simulink model "fin_long_curs2"  (R2019a)
settings: Solver=VariableStepAuto  StartTime=0.0  StopTime=100  RelTol=1e-3
values from neighbouring files (symbols this model uses):
  c1 = 743    [scr1.m]
  C_d1 = c_dl1    [scr1.m]
  C_d3 = c_dl_3    [scr1.m]
  C_n1 = c_np1    [scr1.m]
  C_n3 = c_np_3    [scr1.m]
  Ca = 1.19    [scr1.m]
  d12 = conv(d1,d2)    [scr1.m]
  g = 9.8    [scr1.m]
  kr = 0.00026918    [scr1.m]
  M = 1500    [scr1.m]
  n4 = c1/(T*tau1)    (= 3715)    [scr1.m]
  T = 1    [scr1.m]
  tau1 = 0.2    [scr1.m]
  v = 25    [scr1.m]
undefined symbols (not defined in the file or in its folder): c7_dem, c7_num, ci6
settings Model: Creator=hvarol1  LastModifiedBy=Ya
settings DataIOCC: ReturnWorkspaceOutputs=off
settings DebuggingCC: ArithmeticOperatorsInVariantConditions=warning

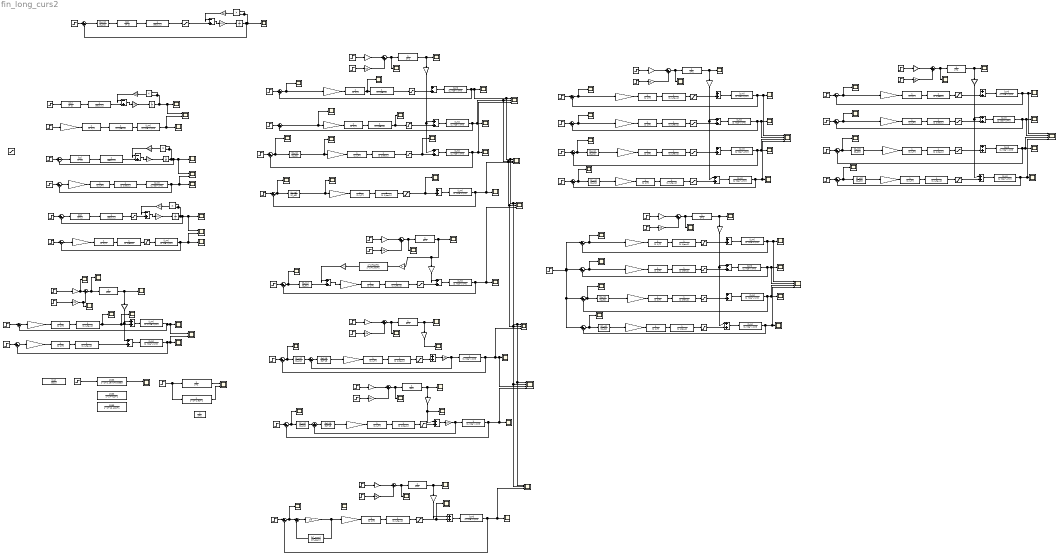
== system fin_long_curs2 ==
  Gain{,1..2,6,30,52} (6 alike) : Gain  Gain=1/M
  Gain{10,16,20,29,32,36,45,55,58} (9 alike) : Gain  Gain=M*g
  Gain{11,17,21,27,33,37,46,56,59} (9 alike) : Gain  Gain=-1
  Gain{3..4,7,12,18,22,28,31,34,38,47,57,60} (13 alike) : Gain  Gain=Ca
  Gain13 : Gain
  Gain14 : Gain  Gain=kr
  Gain{5,8..9,15,19,24..26,35,39..44,48..51,53..54,61..64} (25 alike) : Gain  Gain=c1/(T*tau1)
  Gain23 : Gain  Gain=ci6
  Integrator{,1..3} (4 alike) : Integrator
  Product{1..4} (4 alike) : Product
  Saturation{1,16..19} (5 alike) : Saturate  UpperLimit=16000  LowerLimit=-16000
  Saturation{3..15,20..24} (18 alike) : Saturate  UpperLimit=3500  LowerLimit=-3500
  Saturation2 : Saturate  UpperLimit=10000  LowerLimit=-10000
  Scope{1..4,6..10,12..19,21..25,27,29,32..34,36..41,43..48,50..54,56..64,66..75,77..79,81..93,95..96} (81 alike) : Scope
  Scope{5,11,28,30,35,42} (6 alike) : Scope  NumInputPorts=2
  Scope{20,26,31,49,55} (5 alike) : Scope  NumInputPorts=3
  Scope{65,76,80,94} (4 alike) : Scope  NumInputPorts=4
  Step{,3,9,38} (4 alike) : Step  SampleTime=0
  Step{1..2,4..5,7,10,13,16..19,24..27,30..32,35..37,39..40} (23 alike) : Step  After=25  SampleTime=0
  Step{6,11,14,22,28,33,41,43} (8 alike) : Step  After=100  SampleTime=0
  Step{8,12,15,23,29,34,42,44} (8 alike) : Step  After=0.1  SampleTime=0
  Step20 : Step  Time=300  After=100  SampleTime=0
  Step21 : Step  Time=300  After=0.1  SampleTime=0
  Step45 : Step  Time=50  Before=25  After=35  SampleTime=0
  Sum{1..2,7,28} (4 alike) : Sum  Inputs=|-+
  Sum{8,10,12..14,16,18,20,22..23,25,29..30,32,34,36,38..39,41..42,44,46,48,50,52,54,56,58..59,61,63,65} (32 alike) : Sum  Inputs=|++
  Sum{3..6,9,11,15,17,19,21,24,26..27,31,33,35,37,40,43,45,47,49,51,53,55,57,60,62,64,66} (30 alike) : Sum  Inputs=|+-
  Transfer Fcn{1,7,20,33,60,67,98,108,112} (9 alike) : TransferFcn  Numerator=[C_n1]  Denominator=[C_d1]
  Transfer Fcn{2,4,10,52} (4 alike) : TransferFcn  Denominator=[tau1 1]
  Transfer Fcn100 : TransferFcn  Numerator=[6 18]  Denominator=[5 15]
  Transfer Fcn{6,21,28,39,46,48,53,80,99,101} (10 alike) : TransferFcn  Denominator=[1 1]
  Transfer Fcn{11,14,17,26,30,37,40,49,54,57,61,64,69,71,74,77,81,84,88,92,95,102,105,109,113} (25 alike) : TransferFcn  Denominator=[1 1/T]
  Transfer Fcn{12,15,18,31,34,38,44,50,55,58,62,65,70,72,75,78,82,85,89,93,96,103,106,110,114} (25 alike) : TransferFcn  Denominator=[1 1/tau1]
  Transfer Fcn{16,19,35,45,56,59,63,66,68,73,76,79,83,86,90,94,104,107,111,115} (20 alike) : TransferFcn  Numerator=[1/M]  Denominator=[1 ((Ca*v)/M)]
  Transfer Fcn13 : TransferFcn  Numerator=[1/M]  Denominator=[1 (Ca*v/M)]
  Transfer Fcn22 : TransferFcn  Numerator=[1 6 5]  Denominator=[1 1.8 1]
  Transfer Fcn23 : TransferFcn  Numerator=[1583]  Denominator="[1 2.167  0.8333]"
  Transfer Fcn24 : TransferFcn  Numerator=[n4]  Denominator=[d12]
  Transfer Fcn25 : TransferFcn  Numerator=[1583]  Denominator="[1 41  1]"
  Transfer Fcn27 : TransferFcn  Numerator=[1583]  Denominator="[1 12.48  1]"
  Transfer Fcn29 : TransferFcn  Denominator=[1 1.8 1]
  Transfer Fcn{3,5,9,51} (4 alike) : TransferFcn  Numerator=[c1]  Denominator=[T 1]
  Transfer Fcn32 : TransferFcn  Denominator=[1 ((Ca*v)/M)]
  Transfer Fcn36 : TransferFcn  Numerator=[1/M]  Denominator=[1 (2*Ca*v/M)]
  Transfer Fcn41 : TransferFcn  Numerator=[1/M]  Denominator=[1 (Ca*v/M)]
  Transfer Fcn42 : TransferFcn  Numerator=[6 18]  Denominator=[5 15]
  Transfer Fcn43 : TransferFcn  Numerator=[1 0]  Denominator=[1 1]
  Transfer Fcn47 : TransferFcn  Numerator=[c7_num]  Denominator=[c7_dem]
  Transfer Fcn8 : TransferFcn  Numerator=[C_n3]  Denominator=[C_d3]
  Transfer Fcn87 : TransferFcn  Numerator=[C_n3]  Denominator=[C_d3]
  Transfer Fcn91 : TransferFcn  Numerator=[C_n3]  Denominator=[C_d3]
  Transfer Fcn97 : TransferFcn  Denominator=[1 ((Ca*v)/M)]
  wires:
  Transfer Fcn3/1 -> Transfer Fcn4/1
  Step7/1 -> Sum5/1
  Gain6/1 -> Integrator/1
  Sum7/1 -> Gain6/1
  Product1/1 -> Gain7/1
  Integrator/1 -> Scope28/1, Scope12/1, Sum5/2, Product1/2, Product1/1
  Gain7/1 -> Sum7/1
  Sum1/1 -> Gain2/1
  Product2/1 -> Gain4/1
  Transfer Fcn9/1 -> Transfer Fcn10/1
  Transfer Fcn10/1 -> Sum1/2
  Gain4/1 -> Sum1/1
  Gain2/1 -> Integrator1/1
  Integrator1/1 -> Product2/1, Product2/2, Scope11/1, Scope2/1
  Step3/1 -> Transfer Fcn9/1
  Gain5/1 -> Transfer Fcn14/1
  Transfer Fcn14/1 -> Transfer Fcn15/1
  Sum6/1 -> Gain5/1
  Step4/1 -> Sum6/1
  Sum5/1 -> Transfer Fcn3/1
  Transfer Fcn34/1 -> Sum18/2
  Transfer Fcn38/1 -> Scope38/1, Sum20/2, Scope37/1
  Sum20/1 -> Transfer Fcn36/1
  Sum19/1 -> Gain25/1
  Transfer Fcn36/1 -> Scope35/1, Scope34/1, Sum21/2
  Step18/1 -> Sum19/1
  Gain26/1 -> Transfer Fcn37/1
  Sum18/1 -> Transfer Fcn35/1
  Step19/1 -> Sum21/1
  Transfer Fcn35/1 -> Sum19/2, Scope35/2, Scope33/1
  Step20/1 -> Gain28/1
  Gain28/1 -> Scope40/1, Sum22/2
  Gain29/1 -> Scope41/1, Sum22/1
  Sum21/1 -> Gain26/1
  Gain25/1 -> Transfer Fcn26/1
  Transfer Fcn26/1 -> Transfer Fcn34/1
  Gain27/1 -> Sum18/1, Sum20/1
  Step21/1 -> Gain29/1
  Transfer Fcn37/1 -> Transfer Fcn38/1
  Sum22/1 -> Transfer Fcn46/1, Scope39/1
  Transfer Fcn46/1 -> Gain27/1, Scope36/1
  Transfer Fcn68/1 -> Scope11/2, Scope77/1
  Gain53/1 -> Transfer Fcn71/1
  Transfer Fcn71/1 -> Transfer Fcn72/1
  Step38/1 -> Gain53/1
  Gain35/1 -> Transfer Fcn64/1
  Step27/1 -> Sum40/1
  Transfer Fcn65/1 -> Saturation6/1
  Transfer Fcn64/1 -> Scope14/1, Transfer Fcn65/1
  Transfer Fcn66/1 -> Scope80/1, Scope55/1, Scope49/1, Scope31/1, Scope20/1, Scope26/1, Scope15/1, Sum40/2
  Sum39/1 -> Transfer Fcn66/1
  Gain36/1 -> Sum41/1
  Step28/1 -> Gain38/1
  Sum42/1 -> Transfer Fcn73/1
  Transfer Fcn73/1 -> Scope80/2, Scope55/2, Scope49/2, Scope31/2, Scope20/2, Scope26/2, Scope25/1, Sum43/2
  Step30/1 -> Sum43/1
  Transfer Fcn69/1 -> Transfer Fcn70/1
  Gain39/1 -> Transfer Fcn69/1
  Transfer Fcn74/1 -> Transfer Fcn75/1
  Transfer Fcn76/1 -> Scope26/3, Scope27/1, Sum45/2
  Sum44/1 -> Transfer Fcn76/1
  Step31/1 -> Sum45/1
  Gain40/1 -> Transfer Fcn74/1
  Gain37/1 -> Sum44/1, Sum42/1
  Product3/1 -> Gain3/1
  Gain1/1 -> Integrator2/1
  Integrator2/1 -> Scope1/1, Product3/1, Product3/2, Sum4/2
  Sum2/1 -> Gain1/1
  Gain3/1 -> Sum2/1
  Transfer Fcn2/1 -> Saturation1/1
  Transfer Fcn5/1 -> Transfer Fcn2/1
  Step1/1 -> Sum4/1
  Sum4/1 -> Transfer Fcn1/1
  Transfer Fcn1/1 -> Transfer Fcn5/1
  Transfer Fcn72/1 -> Transfer Fcn68/1
  Transfer Fcn13/1 -> Sum6/2, Scope4/1, Scope28/2
  Transfer Fcn70/1 -> Saturation8/1, Scope7/1
  Gain38/1 -> Sum41/2
  Step29/1 -> Gain36/1
  Transfer Fcn7/1 -> Scope9/1, Gain40/1
  Sum45/1 -> Transfer Fcn7/1, Scope8/1
  Sum40/1 -> Gain35/1, Scope13/1
  Saturation8/1 -> Sum42/2
  Sum43/1 -> Scope6/1, Gain39/1
  Saturation6/1 -> Sum39/2
  Transfer Fcn75/1 -> Saturation3/1
  Sum41/1 -> Transfer Fcn6/1, Scope24/1
  Transfer Fcn6/1 -> Gain37/1, Scope23/1
  Saturation3/1 -> Scope10/1, Sum44/2
  Saturation1/1 -> Sum2/2
  Transfer Fcn8/1 -> Scope19/1, Gain8/1
  Saturation4/1 -> Scope16/1, Sum8/2
  Transfer Fcn11/1 -> Transfer Fcn12/1
  Step2/1 -> Sum9/1
  Gain8/1 -> Transfer Fcn11/1
  Transfer Fcn12/1 -> Saturation4/1
  Transfer Fcn16/1 -> Scope20/3, Scope17/1, Sum9/2
  Sum9/1 -> Transfer Fcn8/1, Scope18/1
  Sum8/1 -> Transfer Fcn16/1
  Sum11/1 -> Transfer Fcn20/1, Scope29/1
  Transfer Fcn19/1 -> Scope31/3, Scope22/1, Sum11/2
  Gain9/1 -> Transfer Fcn17/1
  Transfer Fcn18/1 -> Saturation5/1
  Transfer Fcn17/1 -> Transfer Fcn18/1
  Step5/1 -> Sum11/1
  Sum12/1 -> Transfer Fcn21/1, Scope32/1
  Gain12/1 -> Sum12/2
  Step6/1 -> Gain12/1
  Gain10/1 -> Sum12/1
  Step8/1 -> Gain10/1
  Sum13/1 -> Gain9/1
  Transfer Fcn20/1 -> Sum13/2
  Transfer Fcn22/1 -> Gain13/1
  Step/1 -> Transfer Fcn23/1
  Transfer Fcn23/1 -> Scope30/1
  Step9/1 -> Transfer Fcn28/1, Transfer Fcn29/1
  Transfer Fcn28/1 -> Scope42/1
  Transfer Fcn29/1 -> Scope42/2
  Sum10/1 -> Transfer Fcn19/1
  Saturation5/1 -> Sum10/2
  Gain13/1 -> Sum13/1
  Gain14/1 -> Transfer Fcn22/1
  Transfer Fcn21/1 -> Gain11/1, Gain14/1, Scope21/1
  Sum15/1 -> Scope45/1, Transfer Fcn33/1
  Transfer Fcn32/1 -> Scope49/3, Scope80/3, Scope44/1, Sum15/2
  Gain15/1 -> Transfer Fcn30/1
  Sum14/1 -> Gain/1
  Transfer Fcn30/1 -> Transfer Fcn31/1
  Step10/1 -> Sum15/1
  Sum16/1 -> Transfer Fcn39/1, Scope48/1
  Gain18/1 -> Sum16/2
  Step11/1 -> Gain18/1
  Transfer Fcn39/1 -> Scope47/1, Gain17/1
  Gain16/1 -> Sum16/1
  Step12/1 -> Gain16/1
  Gain17/1 -> Scope43/1
  Transfer Fcn33/1 -> Sum17/1
  Transfer Fcn31/1 -> Saturation9/1
  Gain/1 -> Sum17/2, Transfer Fcn32/1
  Sum17/1 -> Transfer Fcn42/1
  Saturation9/1 -> Sum14/2
  Transfer Fcn42/1 -> Gain15/1
  Transfer Fcn45/1 -> Scope55/3, Scope50/1, Sum24/2
  Gain19/1 -> Transfer Fcn40/1
  Transfer Fcn44/1 -> Saturation7/1
  Saturation7/1 -> Scope46/1, Sum23/2
  Sum23/1 -> Transfer Fcn45/1
  Transfer Fcn40/1 -> Transfer Fcn44/1
  Step13/1 -> Sum24/1
  Gain21/1 -> Sum23/1
  Sum25/1 -> Transfer Fcn48/1, Scope54/1
  Transfer Fcn48/1 -> Scope53/1, Gain21/1
  Gain20/1 -> Sum25/1
  Gain22/1 -> Sum25/2
  Step15/1 -> Gain20/1
  Step14/1 -> Gain22/1
  Sum26/1 -> Gain23/1
  Gain23/1 -> Transfer Fcn47/1, Gain19/1
  Transfer Fcn47/1 -> Sum26/2
  Sum24/1 -> Scope51/1, Sum26/1
  Transfer Fcn15/1 -> Transfer Fcn13/1
  Transfer Fcn4/1 -> Sum7/2
  Saturation13/1 -> Sum28/2
  Step16/1 -> Sum27/1
  Sum3/1 -> Transfer Fcn51/1
  Sum27/1 -> Gain24/1
  Integrator3/1 -> Scope5/1, Scope3/1, Sum3/2, Product4/2, Product4/1
  Step17/1 -> Sum3/1
  Transfer Fcn52/1 -> Saturation13/1
  Gain31/1 -> Sum28/1
  Product4/1 -> Gain31/1
  Transfer Fcn49/1 -> Transfer Fcn50/1
  Transfer Fcn51/1 -> Transfer Fcn52/1
  Gain24/1 -> Transfer Fcn49/1
  Gain30/1 -> Integrator3/1
  Saturation12/1 -> Transfer Fcn41/1
  Sum28/1 -> Gain30/1
  Transfer Fcn41/1 -> Sum27/2, Scope56/1, Scope5/2
  Transfer Fcn50/1 -> Saturation12/1
  Sum29/1 -> Transfer Fcn53/1, Scope58/1
  Gain34/1 -> Sum29/2
  Step22/1 -> Gain34/1
  Transfer Fcn53/1 -> Gain33/1, Scope57/1
  Gain32/1 -> Sum29/1
  Step23/1 -> Gain32/1
  Transfer Fcn56/1 -> Sum31/2, Scope61/1, Scope65/1
  Sum30/1 -> Transfer Fcn56/1
  Step24/1 -> Sum31/1
  Gain41/1 -> Transfer Fcn54/1
  Sum31/1 -> Gain41/1, Scope59/1
  Transfer Fcn54/1 -> Transfer Fcn55/1
  Transfer Fcn55/1 -> Saturation10/1
  Saturation10/1 -> Sum30/2
  Transfer Fcn58/1 -> Saturation11/1
  Transfer Fcn57/1 -> Transfer Fcn58/1
  Saturation11/1 -> Sum32/2
  Sum33/1 -> Gain42/1, Scope62/1
  Step25/1 -> Sum33/1
  Gain42/1 -> Transfer Fcn57/1
  Transfer Fcn59/1 -> Sum33/2, Scope64/1, Scope65/2
  Sum32/1 -> Transfer Fcn59/1
  Transfer Fcn60/1 -> Gain43/1
  Saturation14/1 -> Sum34/2
  Transfer Fcn61/1 -> Transfer Fcn62/1
  Step26/1 -> Sum35/1
  Gain43/1 -> Transfer Fcn61/1
  Transfer Fcn62/1 -> Saturation14/1
  Transfer Fcn63/1 -> Sum35/2, Scope66/1, Scope65/3
  Sum35/1 -> Transfer Fcn60/1, Scope67/1
  Sum34/1 -> Transfer Fcn63/1
  Gain44/1 -> Transfer Fcn77/1
  Step32/1 -> Sum37/1
  Transfer Fcn78/1 -> Saturation15/1
  Sum36/1 -> Transfer Fcn79/1
  Transfer Fcn77/1 -> Transfer Fcn78/1
  Saturation15/1 -> Sum36/2
  Transfer Fcn79/1 -> Sum37/2, Scope65/4, Scope60/1
  Transfer Fcn67/1 -> Gain44/1
  Sum37/1 -> Transfer Fcn67/1, Scope63/1
  Gain33/1 -> Sum36/1, Sum32/1
  Sum53/1 -> Transfer Fcn91/1, Scope74/1
  Saturation19/1 -> Sum52/2
  Transfer Fcn92/1 -> Transfer Fcn93/1
  Transfer Fcn94/1 -> Sum53/2, Scope76/4, Scope71/1
  Sum52/1 -> Transfer Fcn94/1
  Step39/1 -> Sum53/1
  Gain50/1 -> Transfer Fcn88/1
  Transfer Fcn89/1 -> Saturation18/1
  Saturation17/1 -> Sum48/2
  Sum50/1 -> Transfer Fcn90/1
  Sum51/1 -> Transfer Fcn87/1, Scope79/1
  Transfer Fcn88/1 -> Transfer Fcn89/1
  Saturation16/1 -> Sum46/2
  Transfer Fcn82/1 -> Saturation16/1
  Transfer Fcn81/1 -> Transfer Fcn82/1
  Sum47/1 -> Gain48/1, Scope70/1
  Step35/1 -> Sum47/1
  Gain48/1 -> Transfer Fcn81/1
  Gain51/1 -> Transfer Fcn92/1
  Transfer Fcn83/1 -> Sum47/2, Scope72/1, Scope76/1
  Step37/1 -> Sum51/1
  Transfer Fcn84/1 -> Transfer Fcn85/1
  Gain46/1 -> Sum52/1, Sum48/1
  Gain45/1 -> Sum38/1
  Step33/1 -> Gain47/1
  Gain47/1 -> Sum38/2
  Transfer Fcn80/1 -> Gain46/1, Scope68/1
  Sum38/1 -> Transfer Fcn80/1, Scope69/1
  Transfer Fcn93/1 -> Saturation19/1
  Saturation18/1 -> Sum50/2
  Transfer Fcn90/1 -> Sum51/2, Scope78/1, Scope76/3
  Transfer Fcn91/1 -> Gain51/1
  Transfer Fcn87/1 -> Gain50/1
  Sum48/1 -> Transfer Fcn86/1
  Transfer Fcn86/1 -> Sum49/2, Scope75/1, Scope76/2
  Gain49/1 -> Transfer Fcn84/1
  Transfer Fcn85/1 -> Saturation17/1
  Sum46/1 -> Transfer Fcn83/1
  Sum49/1 -> Gain49/1, Scope73/1
  Step36/1 -> Sum49/1
  Step34/1 -> Gain45/1
  Gain11/1 -> Sum10/1
  Sum57/1 -> Transfer Fcn100/1
  Transfer Fcn100/1 -> Gain54/1
  Saturation20/1 -> Sum54/2
  Gain52/1 -> Sum57/2, Transfer Fcn97/1
  Transfer Fcn95/1 -> Transfer Fcn96/1
  Sum54/1 -> Gain52/1
  Transfer Fcn97/1 -> Scope80/4, Scope82/1, Sum55/2
  Gain54/1 -> Transfer Fcn95/1
  Sum55/1 -> Scope83/1, Transfer Fcn98/1
  Transfer Fcn98/1 -> Sum57/1
  Sum56/1 -> Transfer Fcn99/1, Scope85/1
  Transfer Fcn99/1 -> Scope84/1, Gain56/1
  Gain55/1 -> Sum56/1
  Gain57/1 -> Sum56/2
  Step42/1 -> Gain55/1
  Step41/1 -> Gain57/1
  Gain56/1 -> Sum54/1, Scope81/1
  Step40/1 -> Sum55/1
  Transfer Fcn96/1 -> Saturation20/1
  Saturation24/1 -> Sum65/2
  Sum62/1 -> Gain62/1, Scope91/1
  Transfer Fcn115/1 -> Sum66/2, Scope94/4, Scope89/1
  Transfer Fcn113/1 -> Transfer Fcn114/1
  Sum66/1 -> Transfer Fcn112/1, Scope92/1
  Sum63/1 -> Transfer Fcn111/1
  Transfer Fcn108/1 -> Gain63/1
  Gain62/1 -> Transfer Fcn105/1
  Gain63/1 -> Transfer Fcn109/1
  Sum61/1 -> Transfer Fcn107/1
  Gain61/1 -> Transfer Fcn102/1
  Transfer Fcn102/1 -> Transfer Fcn103/1
  Transfer Fcn104/1 -> Sum60/2, Scope90/1, Scope94/1
  Gain58/1 -> Sum58/1
  Sum60/1 -> Gain61/1, Scope88/1
  Saturation21/1 -> Sum59/2
  Gain64/1 -> Transfer Fcn113/1
  Gain59/1 -> Sum65/1, Sum61/1
  Transfer Fcn101/1 -> Gain59/1, Scope86/1
  Transfer Fcn103/1 -> Saturation21/1
  Step45/1 -> Sum64/1, Sum66/1, Sum62/1, Sum60/1
  Sum65/1 -> Transfer Fcn115/1
  Transfer Fcn107/1 -> Sum62/2, Scope93/1, Scope94/2
  Transfer Fcn112/1 -> Gain64/1
  Transfer Fcn109/1 -> Transfer Fcn110/1
  Step43/1 -> Gain60/1
  Sum59/1 -> Transfer Fcn104/1
  Transfer Fcn105/1 -> Transfer Fcn106/1
  Transfer Fcn110/1 -> Saturation23/1
  Transfer Fcn111/1 -> Sum64/2, Scope95/1, Scope94/3
  Saturation23/1 -> Sum63/2
  Sum64/1 -> Transfer Fcn108/1, Scope96/1
  Saturation22/1 -> Sum61/2
  Gain60/1 -> Sum58/2
  Transfer Fcn106/1 -> Saturation22/1
  Sum58/1 -> Transfer Fcn101/1, Scope87/1
  Step44/1 -> Gain58/1
  Transfer Fcn114/1 -> Saturation24/1
